simulink model "Medusa_Model_20130803"  (Simulink 10.1)
settings: Solver=ode45  StartTime=0.0  StopTime=720  RelTol=1e-3  EnableMultiTasking=on
InitFcn:
  | Ts=0.2;
  | 
  | %Kp=45;
  | %Kd=110;
  | Ki=0;
  | Ksat=Inf;
settings Model: Creator=JorgeRibeiro  LastModifiedBy=thomas
settings DataIOCC: LimitDataPoints=on  SignalLoggingSaveFormat=ModelDataLogs
settings OptimizationCC: ExpressionDepthLimit=2147483647
settings DebuggingCC: SolverPrmCheckMsg=warning  FcnCallInpInsideContextMsg=warning  StateNameClashWarn=warning
settings SFSimCC: SimParseCustomCode=off

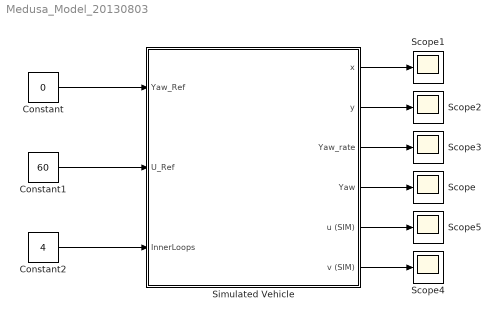
== system Medusa_Model_20130803 ==
  Constant : Constant  Value=0
  Constant1 : Constant  Value=60
  Constant2 : Constant  Value=4
  Scope{,1..5} (6 alike) : Scope
  Simulated Vehicle : Subsystem
  wires:
  Constant/1 -> Simulated Vehicle/1(Yaw_Ref)
  Constant1/1 -> Simulated Vehicle/2(U_Ref)
  Constant2/1 -> Simulated Vehicle/3(InnerLoops)
  Simulated Vehicle/4(Yaw) -> Scope/1
  Simulated Vehicle/1(x) -> Scope1/1
  Simulated Vehicle/3(Yaw_rate) -> Scope3/1
  Simulated Vehicle/2(y) -> Scope2/1
  Simulated Vehicle/5(u (SIM)) -> Scope5/1
  Simulated Vehicle/6(v (SIM)) -> Scope4/1

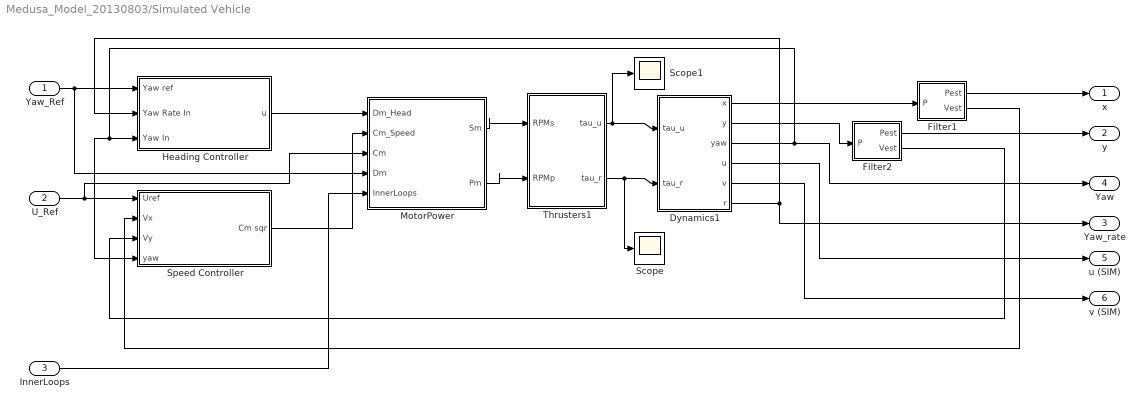
== system Medusa_Model_20130803/Simulated Vehicle ==
  Yaw_Ref : Inport
  U_Ref : Inport  Port=2
  InnerLoops : Inport  Port=3
  Dynamics1 : Subsystem  mask{x0=0, y0=0, yaw0=0, u0=0, v0=0, r0=0, dist_u=0, dist_v=0, dist_r=0, Vcx=0, Vcy=0}
      mask prompts: dist_u "Disturbance in u"; dist_v "Disturbance in v"; dist_r "Disturbance in r"; Vcx "Current x"; Vcy "Current y"
  Filter1 : Subsystem
  Filter2 : Subsystem
  Heading Controller : Subsystem  mask{Kp=45, Kd=110}
  MotorPower : MATLAB Function  TreatAsAtomicUnit=on
  Scope : Scope
  Scope1 : Scope
  "Speed Controller " : Subsystem  mask{Kpu=60, Kiu=2, KSat=60}
      mask prompts: Kpu "Kp"; Kiu "Ki"; KSat "Common Mode Saturation"
  Thrusters1 : Subsystem
  x : Outport
  y : Outport  Port=2
  Yaw_rate : Outport  Port=3
  Yaw : Outport  Port=4
  u (SIM) : Outport  Port=5
  v (SIM) : Outport  Port=6
  wires:
  Thrusters1/1(tau_u) -> Dynamics1/1(tau_u), Scope1/1
  Thrusters1/2(tau_r) -> Scope/1, Dynamics1/2(tau_r)
  Dynamics1/1(x) -> Filter1/1(P)
  Dynamics1/2(y) -> Filter2/1(P)
  Dynamics1/3(yaw) -> Heading Controller/3(Yaw In), "Speed Controller "/4(yaw), Yaw/1
  MotorPower/1(Sm) -> Thrusters1/1(RPMs)
  MotorPower/2(Pm) -> Thrusters1/2(RPMp)
  Dynamics1/6(r) -> Heading Controller/2(Yaw Rate In), Yaw_rate/1
  Filter1/2(Vest) -> "Speed Controller "/2(Vx)
  Filter2/2(Vest) -> "Speed Controller "/3(Vy)
  "Speed Controller "/1(Cm sqr) -> MotorPower/2(Cm_Speed)
  Yaw_Ref/1 -> MotorPower/4(Dm), Heading Controller/1(Yaw ref)
  Filter1/1(Pest) -> x/1
  Filter2/1(Pest) -> y/1
  U_Ref/1 -> MotorPower/3(Cm), "Speed Controller "/1(Uref)
  Heading Controller/1(u) -> MotorPower/1(Dm_Head)
  InnerLoops/1 -> MotorPower/5(InnerLoops)
  Dynamics1/4(u) -> u (SIM)/1
  Dynamics1/5(v) -> v (SIM)/1

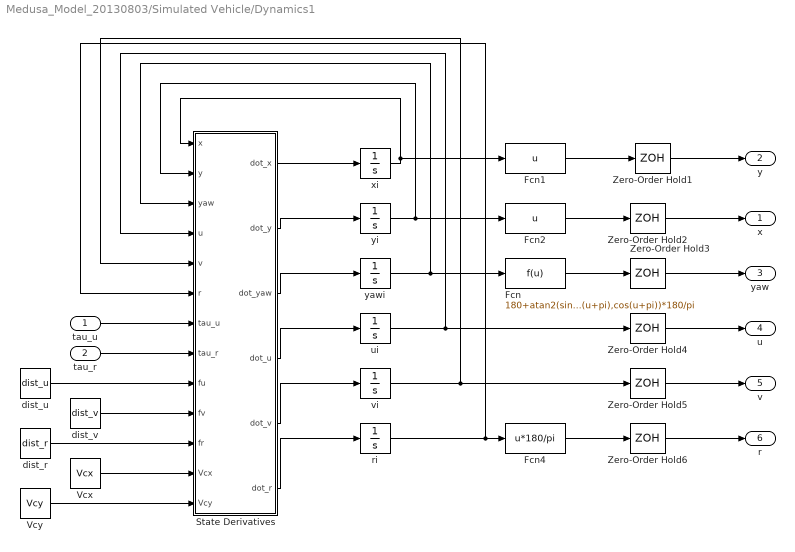
== system Medusa_Model_20130803/Simulated Vehicle/Dynamics1 ==
  tau_u : Inport
  tau_r : Inport  Port=2
  Fcn : Fcn  Expr=180+atan2(sin(u+pi),cos(u+pi))*180/pi
  Fcn1 : Fcn  Expr=u
  Fcn2 : Fcn  Expr=u
  Fcn4 : Fcn  Expr=u*180/pi
  State Derivatives : MATLAB Function  TreatAsAtomicUnit=on
  Vcx : Constant  Value=Vcx
  Vcy : Constant  Value=Vcy
  Zero-Order Hold{1..6} (6 alike) : ZeroOrderHold  SampleTime=0.2
  dist_r : Constant  Value=dist_r
  dist_u : Constant  Value=dist_u
  dist_v : Constant  Value=dist_v
  ri : Integrator  InitialCondition=r0
  ui : Integrator  InitialCondition=u0
  vi : Integrator  InitialCondition=v0
  xi : Integrator  InitialCondition=y0
  yawi : Integrator  InitialCondition=yaw0
  yi : Integrator  InitialCondition=x0
  x : Outport
  y : Outport  Port=2
  yaw : Outport  Port=3
  u : Outport  Port=4
  v : Outport  Port=5
  r : Outport  Port=6
  wires:
  Fcn4/1 -> Zero-Order Hold6/1
  State Derivatives/1(dot_x) -> xi/1
  State Derivatives/2(dot_y) -> yi/1
  State Derivatives/3(dot_yaw) -> yawi/1
  State Derivatives/4(dot_u) -> ui/1
  State Derivatives/5(dot_v) -> vi/1
  State Derivatives/6(dot_r) -> ri/1
  tau_u/1 -> State Derivatives/7(tau_u)
  yi/1 -> State Derivatives/2(y), Fcn2/1
  xi/1 -> State Derivatives/1(x), Fcn1/1
  yawi/1 -> Fcn/1, State Derivatives/3(yaw)
  ui/1 -> State Derivatives/4(u), Zero-Order Hold4/1
  ri/1 -> Fcn4/1, State Derivatives/6(r)
  vi/1 -> State Derivatives/5(v), Zero-Order Hold5/1
  tau_r/1 -> State Derivatives/8(tau_r)
  dist_u/1 -> State Derivatives/9(fu)
  dist_v/1 -> State Derivatives/10(fv)
  dist_r/1 -> State Derivatives/11(fr)
  Fcn/1 -> Zero-Order Hold3/1
  Vcx/1 -> State Derivatives/12(Vcx)
  Vcy/1 -> State Derivatives/13(Vcy)
  Fcn1/1 -> Zero-Order Hold1/1
  Fcn2/1 -> Zero-Order Hold2/1
  Zero-Order Hold1/1 -> y/1
  Zero-Order Hold2/1 -> x/1
  Zero-Order Hold3/1 -> yaw/1
  Zero-Order Hold4/1 -> u/1
  Zero-Order Hold5/1 -> v/1
  Zero-Order Hold6/1 -> r/1

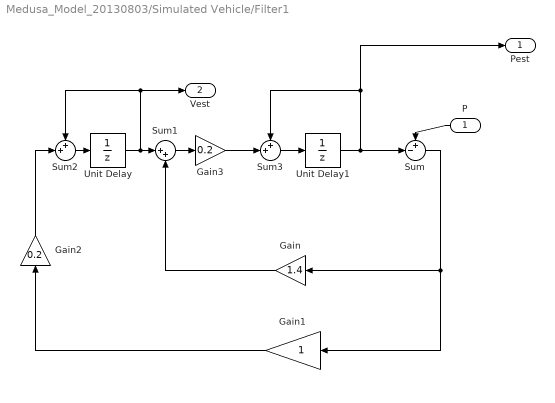
== system Medusa_Model_20130803/Simulated Vehicle/Filter1 ==
  P : Inport
  Gain : Gain  Gain=1.4
  Gain1 : Gain
  Gain2 : Gain  Gain=0.2
  Gain3 : Gain  Gain=0.2
  Sum : Sum  Inputs=+-|
  Sum1 : Sum  Inputs=|++
  Sum2 : Sum  Inputs=++|
  Sum3 : Sum  Inputs=++|
  Unit Delay : UnitDelay  SampleTime=-1
  Unit Delay1 : UnitDelay  SampleTime=-1
  Pest : Outport
  Vest : Outport  Port=2
  wires:
  Sum3/1 -> Unit Delay1/1
  Unit Delay1/1 -> Pest/1, Sum3/1, Sum/2
  Gain3/1 -> Sum3/2
  Gain2/1 -> Sum2/2
  Sum2/1 -> Unit Delay/1
  P/1 -> Sum/1
  Gain1/1 -> Gain2/1
  Unit Delay/1 -> Vest/1, Sum2/1, Sum1/1
  Gain/1 -> Sum1/2
  Sum/1 -> Gain1/1, Gain/1
  Sum1/1 -> Gain3/1

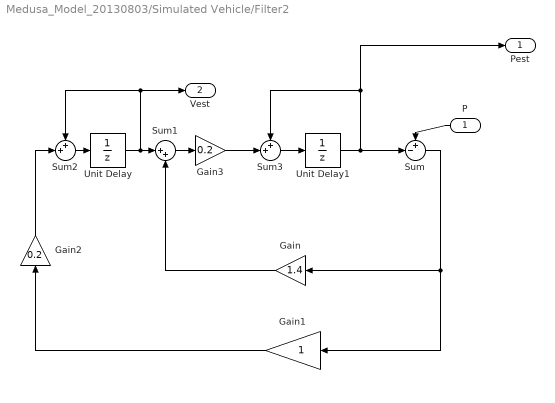
== system Medusa_Model_20130803/Simulated Vehicle/Filter2 ==
  P : Inport
  Gain : Gain  Gain=1.4
  Gain1 : Gain
  Gain2 : Gain  Gain=0.2
  Gain3 : Gain  Gain=0.2
  Sum : Sum  Inputs=+-|
  Sum1 : Sum  Inputs=|++
  Sum2 : Sum  Inputs=++|
  Sum3 : Sum  Inputs=++|
  Unit Delay : UnitDelay  SampleTime=-1
  Unit Delay1 : UnitDelay  SampleTime=-1
  Pest : Outport
  Vest : Outport  Port=2
  wires:
  Sum1/1 -> Gain3/1
  Sum/1 -> Gain/1, Gain1/1
  Gain/1 -> Sum1/2
  Unit Delay/1 -> Sum1/1, Sum2/1, Vest/1
  Gain1/1 -> Gain2/1
  P/1 -> Sum/1
  Sum2/1 -> Unit Delay/1
  Gain2/1 -> Sum2/2
  Gain3/1 -> Sum3/2
  Unit Delay1/1 -> Sum/2, Sum3/1, Pest/1
  Sum3/1 -> Unit Delay1/1

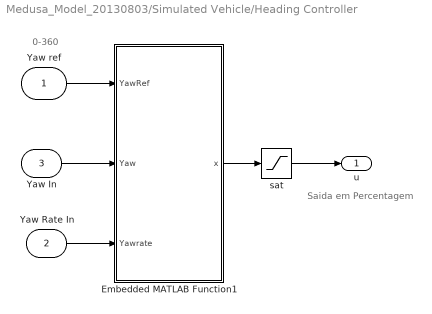
== system Medusa_Model_20130803/Simulated Vehicle/Heading Controller ==
  note: 0-360
  note: Saida em Percentagem
  Yaw ref : Inport  SampleTime=Ts
  Yaw Rate In : Inport  Port=2  SampleTime=Ts
  Yaw In : Inport  Port=3
  Embedded MATLAB Function1 : MATLAB Function  TreatAsAtomicUnit=on
  sat : Saturate  UpperLimit=Inf  LowerLimit=-Inf  SampleTime=Ts
  u : Outport
  wires:
  Yaw ref/1 -> Embedded MATLAB Function1/1(YawRef)
  Embedded MATLAB Function1/1(x) -> sat/1
  Yaw In/1 -> Embedded MATLAB Function1/2(Yaw)
  Yaw Rate In/1 -> Embedded MATLAB Function1/3(Yawrate)
  sat/1 -> u/1

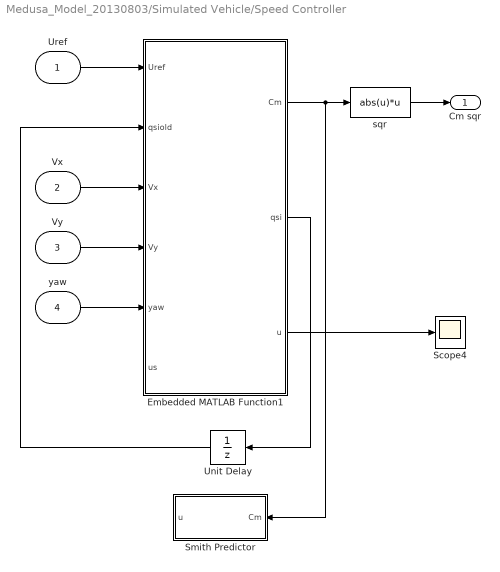
== system Medusa_Model_20130803/Simulated Vehicle/Speed Controller  ==
  Uref : Inport
  Vx : Inport  Port=2
  Vy : Inport  Port=3
  yaw : Inport  Port=4
  Embedded MATLAB Function1 : MATLAB Function  TreatAsAtomicUnit=on
  Scope4 : Scope
  Smith Predictor : Subsystem
  Unit Delay : UnitDelay  SampleTime=0.2
  sqr : Fcn  Expr=abs(u)*u
  Cm sqr : Outport
  wires:
  Embedded MATLAB Function1/3(u) -> Scope4/1
  yaw/1 -> Embedded MATLAB Function1/5(yaw)
  Vy/1 -> Embedded MATLAB Function1/4(Vy)
  Vx/1 -> Embedded MATLAB Function1/3(Vx)
  Embedded MATLAB Function1/1(Cm) -> Smith Predictor/1(Cm), sqr/1
  Uref/1 -> Embedded MATLAB Function1/1(Uref)
  Embedded MATLAB Function1/2(qsi) -> Unit Delay/1
  Unit Delay/1 -> Embedded MATLAB Function1/2(qsiold)
  sqr/1 -> Cm sqr/1

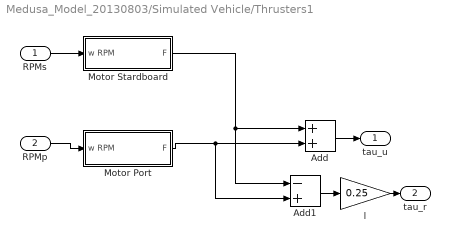
== system Medusa_Model_20130803/Simulated Vehicle/Thrusters1 ==
  RPMs : Inport
  RPMp : Inport  Port=2
  Add : Sum
  Add1 : Sum  Inputs=-+
  Motor Port : Subsystem  mask{K0=7.2115, tau=0.346, eta=4/(1500^2)}
      mask prompts: tau "Atraso do Motor"; eta "Constante de conversao W-F"
  Motor Stardboard : Subsystem  mask{K0=7.2115, tau=0.346, eta=4/(1500^2)}
      mask prompts: tau "Atraso do Motor"; eta "Constante de conversao W-F"
  l : Gain  Gain=0.25
  tau_u : Outport
  tau_r : Outport  Port=2
  wires:
  Add1/1 -> l/1
  RPMs/1 -> Motor Stardboard/1(w RPM)
  Add/1 -> tau_u/1
  RPMp/1 -> Motor Port/1(w RPM)
  l/1 -> tau_r/1
  Motor Port/1(F) -> Add/2, Add1/2
  Motor Stardboard/1(F) -> Add/1, Add1/1

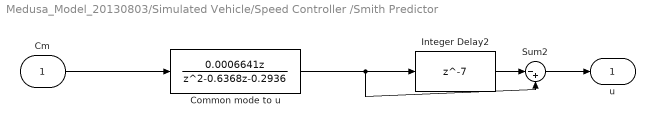
== system Medusa_Model_20130803/Simulated Vehicle/Speed Controller /Smith Predictor ==
  Cm : Inport
  Common mode to u : DiscreteTransferFcn  Numerator=[0.0006641 0]  Denominator=[1 -0.6368 -0.2936]  SampleTime=0.2
  Integer Delay2 : Delay  DelayLength=7  SampleTime=0.2
  Sum2 : Sum  Inputs=|-+
  u : Outport
  wires:
  Cm/1 -> Common mode to u/1
  Common mode to u/1 -> Integer Delay2/1, Sum2/2
  Integer Delay2/1 -> Sum2/1
  Sum2/1 -> u/1

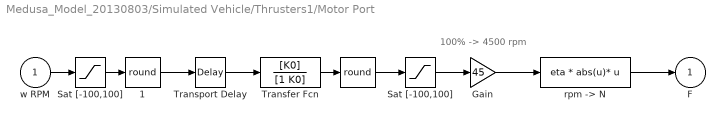
== system Medusa_Model_20130803/Simulated Vehicle/Thrusters1/Motor Port ==
  note: 100% -> 4500 rpm
  w RPM : Inport
  "  " : Rounding  Operator=round
  "  1" : Rounding  Operator=round
  Gain : Gain  Gain=45
  Sat [-100,100] : Saturate  UpperLimit=100  LowerLimit=-100
  "Sat [-100,100] " : Saturate  UpperLimit=100  LowerLimit=-100
  Transfer Fcn : TransferFcn  Numerator=[K0]  Denominator=[1 K0]
  Transport Delay : TransportDelay  DelayTime=tau
  "rpm -> N" : Fcn  Expr=eta * abs(u)* u
  F : Outport
  wires:
  Transfer Fcn/1 -> "  "/1
  Transport Delay/1 -> Transfer Fcn/1
  "  1"/1 -> Transport Delay/1
  "  "/1 -> "Sat [-100,100] "/1
  "rpm -> N"/1 -> F/1
  Sat [-100,100]/1 -> "  1"/1
  Gain/1 -> "rpm -> N"/1
  w RPM/1 -> Sat [-100,100]/1
  "Sat [-100,100] "/1 -> Gain/1

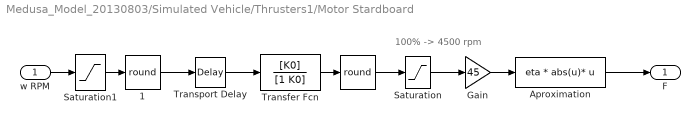
== system Medusa_Model_20130803/Simulated Vehicle/Thrusters1/Motor Stardboard ==
  note: 100% -> 4500 rpm
  w RPM : Inport
  "  " : Rounding  Operator=round
  "  1" : Rounding  Operator=round
  Aproximation : Fcn  Expr=eta * abs(u)* u
  Gain : Gain  Gain=45
  Saturation : Saturate  UpperLimit=100  LowerLimit=-100
  Saturation1 : Saturate  UpperLimit=100  LowerLimit=-100
  Transfer Fcn : TransferFcn  Numerator=[K0]  Denominator=[1 K0]
  Transport Delay : TransportDelay  DelayTime=tau
  F : Outport
  wires:
  Transfer Fcn/1 -> "  "/1
  Transport Delay/1 -> Transfer Fcn/1
  "  1"/1 -> Transport Delay/1
  "  "/1 -> Saturation/1
  Aproximation/1 -> F/1
  Saturation1/1 -> "  1"/1
  Gain/1 -> Aproximation/1
  w RPM/1 -> Saturation1/1
  Saturation/1 -> Gain/1

== matlab function Simulated Vehicle/Dynamics1/State Derivatives ==
  data: x input double; y input double; yaw input double; u input double; v input double; r input double; tau_u input double; dot_x output double; tau_r input double; dot_y output double; dot_yaw output double; dot_u output double; dot_v output double; dot_r output double; fu input double; fv input double; fr input double; Vcx input double; Vcy input double
function [dot_x,dot_y,dot_yaw,dot_u,dot_v,dot_r] = fcn(x,y,yaw,u,v,r,tau_u,tau_r,fu,fv,fr, Vcx, Vcy)
%state = [x, y, yaw, u, v, r]

% %%%%%% Coefficients
% mass = 17.0;
% I_z = 4.14;
% X_dot_u = -20;
% Y_dot_v = -1.3175;
% N_dot_r =  -8.69;
% X_u = -0.2;
% Y_v = -55.117;
% N_r = -4.14;
% X_uu = -25; 
% Y_vv = -101.2776;
% N_rr = -6.23;

%%%%%% Coefficients
mass = 17.0;
I_z = 1;
X_dot_u = -20;
Y_dot_v = -30;%-1.3175;
N_dot_r = -8.69;% -0.5;
X_u = -0.2;
Y_v = -50;
N_r = -4.14; %-0.1
X_uu = -25; 
Y_vv = -0.01;%-101.2776;
N_rr = -6.23; %-21

%%%%%% masses
m_u = mass - X_dot_u;
m_v = mass - Y_dot_v;
m_r = I_z - N_dot_r;
m_uv = m_u - m_v;

%%%%%%%%% drag

d_u = -X_u - X_uu*abs(u);
d_v = -Y_v - Y_vv*abs(v);
d_r = -N_r - N_rr*abs(r);

%%%%%%%%% Dynamics

dot_u = 1/m_u*(tau_u + m_v*v*r - d_u*u+fu);
dot_v = 1/m_v*(-m_u*u*r - d_v*v+fv);
dot_r = 1/m_r*(tau_r + m_uv*u*v - d_r*r+fr);

dot_x = u*cos(yaw) - v*sin(yaw) + Vcx;
dot_y = u*sin(yaw) + v*cos(yaw) + Vcy;
dot_yaw = r;

== matlab function Simulated Vehicle/Heading Controller/Embedded MATLAB Function1 ==
  data: YawRef input double; x output double; Yaw input double; Yawrate input double; Kd parameter double; Kp parameter double
function x = controller(YawRef, Yaw, Yawrate, Kd, Kp)
err = ( YawRef- Yaw );
if(err>180) 
     err=err-360;
elseif(err<-180) 
     err=360+err;
end

x=Kp*err-Kd*Yawrate;

== matlab function Simulated Vehicle/MotorPower ==
  data: Dm_Head input double; Sm output double; Pm output double; Cm_Speed input double; Cm input double; Dm input double; InnerLoops input double
function [Sm,Pm] = fcn(Dm_Head, Cm_Speed, Cm, Dm, InnerLoops)
Cm_sqr=0;
Dm_sqr=0;
switch InnerLoops
    case 0
        ; % Don't do anything
    case 1
        Cm_sqr=Cm_Speed;
        Dm_sqr=Dm_Head;
    case 2
        Cm_sqr=Cm*abs(Cm);
        Dm_sqr=Dm_Head;
    case 3
        Cm_sqr=Cm_Speed;
        Dm_sqr=Dm*abs(Dm);
    case 4
        Cm_sqr=Cm*abs(Cm);
        Dm_sqr=Dm*abs(Dm);
    otherwise
end

Pm = round(sqrt(abs(Cm_sqr+Dm_sqr))*sign(Cm_sqr+Dm_sqr));
Sm = round(sqrt(abs(Cm_sqr-Dm_sqr))*sign(Cm_sqr-Dm_sqr));

== matlab function Simulated Vehicle/Speed Controller /Embedded MATLAB Function1 ==
  data: Cm output double; Uref input double; Kpu parameter double; Kiu parameter double; qsiold input double; qsi output double; Vx input double; Vy input double; yaw input double; u output double; us input double; KSat parameter double
function [Cm, qsi, u] = controller(Uref, Kpu,Kiu, qsiold,Vx,Vy,yaw, us, KSat)
u=Vx*sind(yaw)+Vy*cosd(yaw);
err=u-Uref;
qsi=qsiold+err;

Cm=-Kpu*(err+us)-Kiu*qsi;
% Cm =+40*Uref-Kiu*qsi;
% if(t>10)
%     qsi=qsiold+err;
%     Cm =-Kpu*err-Kiu*qsi;
% end
if(abs(Cm) >= KSat)
   Cm = KSat*sign(Cm); 
   qsi = qsiold;
end
